simulink model "ASW_ABS"  (R2025b)
settings: Solver=VariableStepAuto  StartTime=0.0  StopTime=10.0  RelTol=1e-3
undefined symbols (not defined in the file): DiscIntNeverNeededParam, g, m, mu, Rr, slip, v0
settings Model: Creator=WangPuzheng(CNTV-M1)  LastModifiedBy=WangPuzheng(CNTV-M1)
settings HardwareCC: TargetBitPerPointer=64.0  TargetBitPerSizeT=64.0  TargetBitPerPtrDiffT=64.0  TargetLongLongMode=on  TargetIntDivRoundTo=Zero  TargetEndianess=LittleEndian  TargetWordSize=64.0  TargetHWDeviceType=MATLAB Host  ProdEqTarget=off
settings RTWCC: SystemTargetFile=rsim.tlc  GenCodeOnly=on  TemplateMakefile=rsim_default_tmf  Description=Rapid Simulation Target
settings RSimTargetCC: RSIM_SOLVER_SELECTION=UseFixStep  ExtModeTransport=0.0  ExtModeStaticAllocSize=1000000.0  TargetLangStandard=C99 (ISO)  MultiwordLength=2048.0  DynamicStringBufferSize=256.0  PreserveMATLABNamespacesInGeneratedCode=on  SubcomponentCodeInterfacePackaging=Reusable function  InstructionSetFMA=off  OptimizeReductions=off  LogToMDFFile=off

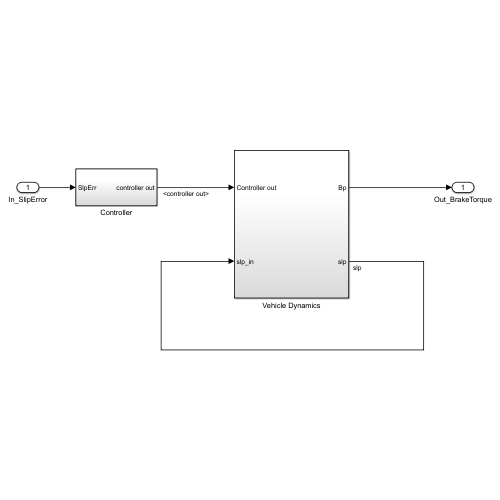
[thumbnail: Simulink's stored preview of the top-level diagram]
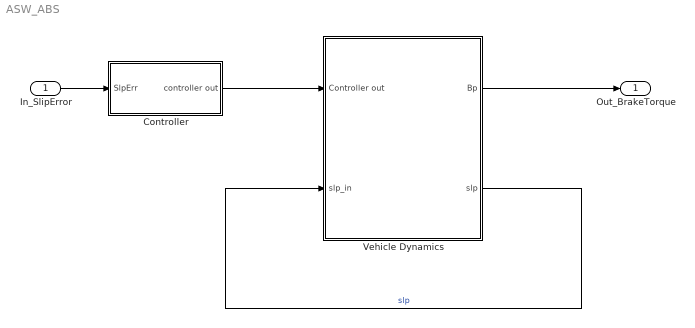
== system ASW_ABS ==
  In_SlipError : Inport
  Controller : Subsystem
  Vehicle Dynamics : Subsystem
  Out_BrakeTorque : Outport
  wires:
  In_SlipError/1 -> Controller/1(SlpErr)
  Controller/1(controller out) -> Vehicle Dynamics/1(Controller out)
  Vehicle Dynamics/2(slp) -> Vehicle Dynamics/2(slp_in)  "slp"
  Vehicle Dynamics/1(Bp) -> Out_BrakeTorque/1

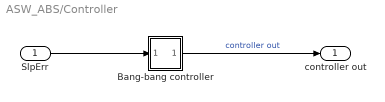
== system ASW_ABS/Controller ==
  SlpErr : Inport
  Bang-bang controller : Subsystem  mask(Sign){}
      mask help: y = sign(x)
      mask Help: Sign Function:\n\t\t\ty = 1 if x > 0\n\t\t\ty = 0 if x = 0\n\t\t\ty = -1 if x < 0
      mask Display: plot(-50,-50,50,50,[-50,50],[0,0],[0,0],[-50,50],[-40,0],[-30,-30],[0,40],[30,30])
  controller out : Outport
  wires:
  Bang-bang controller/1(out_1) -> controller out/1  "controller out"
  SlpErr/1 -> Bang-bang controller/1(in_1)

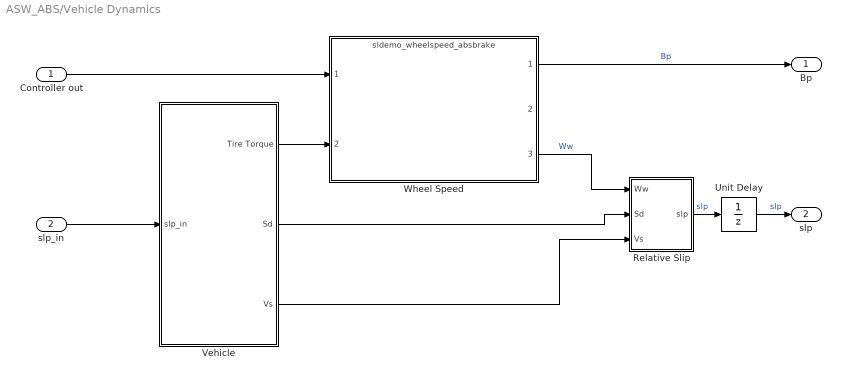
== system ASW_ABS/Vehicle Dynamics ==
  Controller out : Inport
  slp_in : Inport  Port=2
  Relative Slip : Subsystem
  Unit Delay : UnitDelay  SampleTime=-1  HasFrameUpgradeWarning=on
  "Vehicle  " : Subsystem
  Wheel Speed : ModelReference  ModelNameDialog=sldemo_wheelspeed_absbrake.slx  SimulationMode=Normal  ModelReferenceVersion=11.1
  Bp : Outport
  slp : Outport  Port=2
  wires:
  Wheel Speed/3 -> Relative Slip/1(Ww)  "Ww"
  "Vehicle  "/3(Vs) -> Relative Slip/3(Vs)
  "Vehicle  "/1(Tire Torque) -> Wheel Speed/2
  "Vehicle  "/2(Sd) -> Relative Slip/2(Sd)
  Relative Slip/1(slp) -> Unit Delay/1  "slp"
  Controller out/1 -> Wheel Speed/1
  Wheel Speed/1 -> Bp/1  "Bp"
  slp_in/1 -> "Vehicle  "/1(slp_in)
  Unit Delay/1 -> slp/1  "slp"

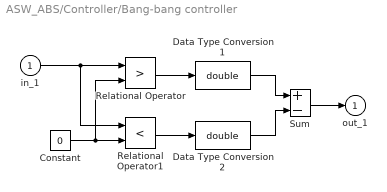
== system ASW_ABS/Controller/Bang-bang controller ==
  in_1 : Inport
  Constant : Constant  Value=0
  Data Type Conversion1 : DataTypeConversion  OutDataTypeStr=double
  Data Type Conversion2 : DataTypeConversion  OutDataTypeStr=double
  Relational Operator : RelationalOperator  Operator=>  OutDataTypeStr=boolean
  Relational Operator1 : RelationalOperator  Operator=<  OutDataTypeStr=boolean
  Sum : Sum  Inputs=+-  InputSameDT=on  SaturateOnIntegerOverflow=on  OutDataTypeStr=Inherit: Same as first input
  out_1 : Outport  InitialOutput=0  VectorParamsAs1DForOutWhenUnconnected=off
  wires:
  Data Type Conversion2/1 -> Sum/2
  Data Type Conversion1/1 -> Sum/1
  Sum/1 -> out_1/1
  Relational Operator/1 -> Data Type Conversion1/1
  Relational Operator1/1 -> Data Type Conversion2/1
  Constant/1 -> Relational Operator/2, Relational Operator1/2
  in_1/1 -> Relational Operator1/1, Relational Operator/1

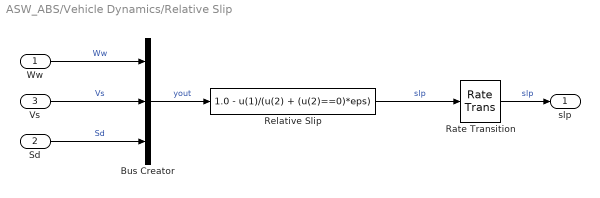
== system ASW_ABS/Vehicle Dynamics/Relative Slip ==
  Ww : Inport
  Sd : Inport  Port=2
  Vs : Inport  Port=3
  Bus Creator : BusCreator  Inputs=3
  Rate Transition : RateTransition  OutPortSampleTimeOpt=Inherit
  Relative Slip : Fcn  Expr=1.0 - u(1)/(u(2) + (u(2)==0)*eps)
  slp : Outport
  wires:
  Bus Creator/1 -> Relative Slip/1  "yout"
  Relative Slip/1 -> Rate Transition/1  "slp"
  Ww/1 -> Bus Creator/1  "Ww"
  Vs/1 -> Bus Creator/2  "Vs"
  Sd/1 -> Bus Creator/3  "Sd"
  Rate Transition/1 -> slp/1  "slp"

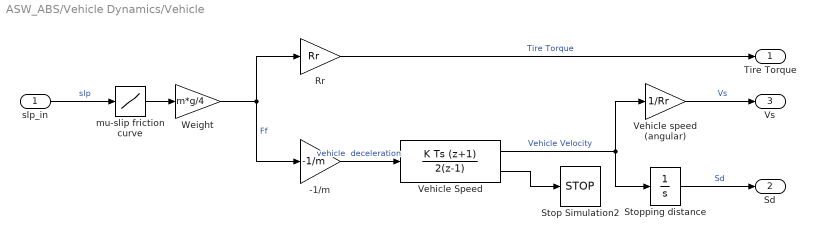
== system ASW_ABS/Vehicle Dynamics/Vehicle   ==
  slp_in : Inport
  -1/m : Gain  Gain=-1/m  SaturateOnIntegerOverflow=on  OutDataTypeStr=Inherit: Same as input  ParamDataTypeStr=Inherit: Same as input
  Rr : Gain  Gain=Rr  SaturateOnIntegerOverflow=on  OutDataTypeStr=Inherit: Same as input  ParamDataTypeStr=Inherit: Same as input
  Stop Simulation2 : Stop
  Stopping distance : Integrator  UpperSaturationLimit=1000  LowerSaturationLimit=0
  Vehicle Speed : DiscreteIntegrator  IntegratorMethod=Integration: Trapezoidal  InitialCondition=v0  SampleTime=-1  LimitOutput=on  UpperSaturationLimit=1000  LowerSaturationLimit=0  ShowSaturationPort=on  ICPrevOutput=DiscIntNeverNeededParam  ICPrevScaledInput=DiscIntNeverNeededParam
  Vehicle speed (angular) : Gain  Gain=1/Rr  SaturateOnIntegerOverflow=on  OutDataTypeStr=Inherit: Same as input  ParamDataTypeStr=Inherit: Same as input
  Weight : Gain  Gain=m*g/4  SaturateOnIntegerOverflow=on  OutDataTypeStr=Inherit: Same as input  ParamDataTypeStr=Inherit: Same as input
  mu-slip friction curve : Lookup_n-D  NumberOfTableDimensions=1  BreakpointsForDimension1=slip  Table=mu  SaturateOnIntegerOverflow=on
  Tire Torque : Outport  Unit=N*m
  Sd : Outport  Port=2  Unit=m
  Vs : Outport  Port=3  Unit=rad/sec
  wires:
  slp_in/1 -> mu-slip friction curve/1  "slp"
  Rr/1 -> Tire Torque/1  "Tire Torque"
  -1/m/1 -> Vehicle Speed/1  "vehicle  deceleration"
  Vehicle speed (angular)/1 -> Vs/1  "Vs"
  Stopping distance/1 -> Sd/1  "Sd"
  Weight/1 -> -1/m/1, Rr/1  "Ff"
  mu-slip friction curve/1 -> Weight/1
  Vehicle Speed/1 -> Vehicle speed (angular)/1, Stopping distance/1  "Vehicle Velocity"
  Vehicle Speed/2 -> Stop Simulation2/1
